simulink model "quadruped_2016"  (R2016a)
settings: Solver=ode23t  SolverMode=SingleTasking  StartTime=0.0  StopTime=8  RelTol=1e-3
values from neighbouring files (symbols this model uses):
  robot = Robot    [quadruped_sim_param.m]
undefined symbols (not defined in the file or in its folder): sigbuilder_block, X, Y, Z
undefined symbols (not defined in the file): plane
libraries: sm_lib x138, nesl_utility x66, simulink x24, Contact_Forces_Lib x12
(part 1 of 5)
settings Model: Creator=krzysiek  LastModifiedBy=krzysiek
settings SolverCC: ZeroCrossAlgorithm=Adaptive
settings DataIOCC: ReturnWorkspaceOutputs=on
settings DebuggingCC: IgnoredZcDiagnostic=none  SFUnexpectedBacktrackingDiag=error  SFNoUnconditionalDefaultTransitionDiag=error
settings SFSimCC: SimUseLocalCustomCode=on
settings RTWCC: RTWUseLocalCustomCode=on
settings GRTTargetCC: TargetLangStandard=C99 (ISO)  GeneratePreprocessorConditionals=Use local settings
settings ConfigComp: CovMetricSettings=dwe  CovHtmlReporting=off  CovSaveCumulativeToWorkspaceVar=off  CovSaveSingleToWorkspaceVar=off  CovExternalEMLEnable=on
settings DiagnosticsConfigSet: SimMechanicsRigidlyBoundBlock=none

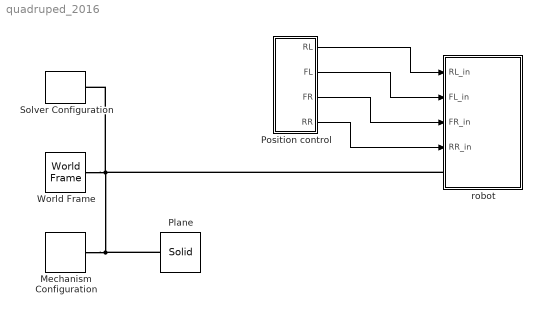
== system quadruped_2016 ==
  Mechanism Configuration : sm_lib/Utilities/Mechanism Configuration  UniformGravity=Constant  GravityVector=[0 0 -9.80665]  GravityUnits=m/s^2  LinearizationDelta=0.001
  "Plane " : sm_lib/Body Elements/Solid  GraphicAmbientColor=[0.15 0.15 0.15 1.0]  BasedOnType=Density  BrickDimensions=plane  BrickDimensionUnits=m  CenterOfMass=[0 0 0]  CenterOfMassUnits=m  GraphicDiffuseColor=[0.5 0.5 0.5]  Density=1000  DensityUnits=kg/m^3  DoExposeReferenceFrame=on  GraphicEmissiveColor=[0.0 0.0 0.0 1.0]  ExportEntireGeometry=off  SerializedFrames=<Frames/>  MarkerShape=Sphere  MarkerSize=10  GraphicType=FromGeometry  InertiaType=CalculateFromGeometry  Mass=1  MassUnits=kg  MomentsOfInertia=[1 1 1]  MomentsOfInertiaUnits=kg*m^2  GraphicOpacity=1.0  ProductsOfInertia=[0 0 0]  ProductsOfInertiaUnits=kg*m^2  GraphicShininess=75  GraphicSpecularColor=[0.5 0.5 0.5 1.0]  GraphicVisPropType=SimpleVisualProperties  GeometryShape=Brick
  Position control : Subsystem
  Solver Configuration : nesl_utility/Solver Configuration  PhysicalDomain=network_engine_domain  SubClassName=solver  LeftPortType=input  RightPortType=generic  Tones=[]  Harmonics=[]  SimulateNoise=off  Profile=off  UseLocalSampling=off  EnableSwitchedLinearOptims=on  FrequencyDomain=off  UseCCode=off  RelTol=0.001  AbsTol=1e-06  MinStep=1e-09  ToWorkspace=off  RevertToSquareIcSolve=off  NumHomotopyIterations=100  PhasorMode=off  PhasorModeNumHarmonics=1  DoDC=off  ResidualTolerance=1e-09  UseLocalSolver=off  LocalSolverChoice=NE_TRAPEZOIDAL_ADVANCER  LocalSolverSampleTime=0.1  DoFixedCost=off  MaxNonlinIter=3  MaxModeIter=2  LinearAlgebra=Sparse  EquationFormulation=NE_TIME_EF  DelaysMemoryBudget=1024  AutomaticFiltering=on  FilteringTimeConstant=0.001  PartitionStorageMethod=AS_NEEDED  PartitionMemoryBudget=1024  PartitionMethod=FAST
  World Frame : sm_lib/Frames and Transforms/World Frame
  robot : Subsystem
  wires:
  Position control/1(RL) -> robot/1(RL_in)
  Position control/2(FL) -> robot/2(FL_in)
  Position control/3(FR) -> robot/3(FR_in)
  Position control/4(RR) -> robot/4(RR_in)
  connections:
  World Frame/RConn1 -- Mechanism Configuration/RConn1 -- "Plane "/RConn1 -- robot/LConn1 -- Solver Configuration/RConn1

== system quadruped_2016/Position control ==
  Constant1 : Constant  Value=robot.FL.hip.joint.base_angle
  Constant2 : Constant  Value=robot.FR.hip.joint.base_angle
  Constant3 : Constant  Value=robot.RR.hip.joint.base_angle
  Constant6 : Constant  Value=robot.RL.hip.joint.base_angle
  Mux{1..4} (4 alike) : Mux  Inputs=3
  Signal Builder : Subsystem  Tag=STV Subsys  LoadFcn=sigbuilder_block('load');  StartFcn=sigbuilder_block('start');  StopFcn=sigbuilder_block('stop');  ClipboardFcn=sigbuilder_block('clipboard');  mask(Sigbuilder block){}
      mask help: Simulink:masks:SigbuilderBlock_MD
      mask init:
      | if ~strcmp(get_param(bdroot(gcbh),'SimulationStatus'),'stopped') tuvar = sigbuilder_block('maskInit'); end
      settings: CopyFcn=sigbuilder_block('copy');  DeleteFcn=sigbuilder_block('delete');  ModelCloseFcn=sigbuilder_block('modelClose');  PreSaveFcn=sigbuilder_block('preSave');  PauseFcn=sigbuilder_block('pause');  ContinueFcn=sigbuilder_block('continue');  NameChangeFcn=sigbuilder_block('namechange');  OpenFcn=sigbuilder_block('open',[1212.63 0 1212.63 628.421 ]);  CloseFcn=sigbuilder_block('close');
      mask Display: plot(0, 0, 100, 100,[2, 2, 32, 32, 2], [68, 8, 8, 68, 68],[32, 2], [38, 38], [32, 19, 2],[53, 60, 44], [32, 17, 17, 2],[16, 16, 31, 31]);txt = getActiveGroup(gcbh);text(2, 100, txt,'verticalAlignment', 'top');
  RL : Outport
  FL : Outport  Port=2
  FR : Outport  Port=3
  RR : Outport  Port=4
  wires:
  Mux2/1 -> RL/1
  Constant6/1 -> Mux2/3  "hip pos"
  Mux1/1 -> FL/1
  Constant1/1 -> Mux1/3  "hip pos"
  Mux3/1 -> FR/1
  Constant2/1 -> Mux3/3  "hip pos"
  Mux4/1 -> RR/1
  Constant3/1 -> Mux4/3  "hip pos"
  Signal Builder/1(Rx) -> Mux2/1, Mux4/1  "x"
  Signal Builder/2(Ry) -> Mux2/2, Mux4/2
  Signal Builder/3(Fx) -> Mux1/1, Mux3/1  "x"
  Signal Builder/4(Fy) -> Mux1/2, Mux3/2  "y"

== system quadruped_2016/robot ==
  RL_in : Inport
  FL_in : Inport  Port=2
  FR_in : Inport  Port=3
  RR_in : Inport  Port=4
  6-DOF Joint1 : sm_lib/Joints/6-DOF Joint  JointMode=Normal  SenseConstraintForce=off  SenseConstraintForceX=off  SenseConstraintForceY=off  SenseConstraintForceZ=off  SenseConstraintTorque=off  SenseConstraintTorqueX=off  SenseConstraintTorqueY=off  SenseConstraintTorqueZ=off  SenseTotalForce=off  SenseTotalForceX=off  SenseTotalForceY=off  SenseTotalForceZ=off  SenseTotalTorque=off  SenseTotalTorqueX=off  SenseTotalTorqueY=off  SenseTotalTorqueZ=off  CompositeWrenchDir=FollowerOnBase  CompositeWrenchFrame=BaseFrame  PxEquilibriumPosition=0  PxEquilibriumPositionUnits=m  PxSpringStiffness=0  PxSpringStiffnessUnits=N/m  PxDampingCoefficient=0  PxDampingCoefficientUnits=N/(m/s)  PxTorqueActuationMode=NoTorque  PxMotionActuationMode=ComputedMotion  PxSensePosition=off  PxSenseVelocity=off  PxSenseAcceleration=off  PxSenseTorqueForce=off  PxSenseLowerLimitTorqueForce=off  PxSenseUpperLimitTorqueForce=off  PxLowerLimitSpecify=off  PxLowerLimitBound=-1  PxLowerLimitBoundUnits=m  PxLowerLimitStiffness=1e6  PxLowerLimitStiffnessUnits=N/m  PxLowerLimitDamping=1e3  PxLowerLimitDampingUnits=N/(m/s)  PxLowerLimitTransitionRegionWidth=1e-4  PxLowerLimitTransitionRegionWidthUnits=m  PxUpperLimitSpecify=off  PxUpperLimitBound=1  PxUpperLimitBoundUnits=m  PxUpperLimitStiffness=1e6  PxUpperLimitStiffnessUnits=N/m  PxUpperLimitDamping=1e3  PxUpperLimitDampingUnits=N/(m/s)  PxUpperLimitTransitionRegionWidth=1e-4  PxUpperLimitTransitionRegionWidthUnits=m  PxPositionTargetSpecify=off  PxPositionTargetPriority=High  PxPositionTargetValue=0  PxPositionTargetValueUnits=m  PxVelocityTargetSpecify=off  PxVelocityTargetPriority=High  PxVelocityTargetValue=0  PxVelocityTargetValueUnits=m/s  PyEquilibriumPosition=0  PyEquilibriumPositionUnits=m  PySpringStiffness=0  PySpringStiffnessUnits=N/m  PyDampingCoefficient=0  PyDampingCoefficientUnits=N/(m/s)  PyTorqueActuationMode=NoTorque  PyMotionActuationMode=ComputedMotion  PySensePosition=off  PySenseVelocity=off  PySenseAcceleration=off  PySenseTorqueForce=off  PySenseLowerLimitTorqueForce=off  PySenseUpperLimitTorqueForce=off  PyLowerLimitSpecify=off  PyLowerLimitBound=-1  PyLowerLimitBoundUnits=m  PyLowerLimitStiffness=1e6  PyLowerLimitStiffnessUnits=N/m  PyLowerLimitDamping=1e3  PyLowerLimitDampingUnits=N/(m/s)  PyLowerLimitTransitionRegionWidth=1e-4  PyLowerLimitTransitionRegionWidthUnits=m  PyUpperLimitSpecify=off  PyUpperLimitBound=1  PyUpperLimitBoundUnits=m  PyUpperLimitStiffness=1e6  PyUpperLimitStiffnessUnits=N/m  PyUpperLimitDamping=1e3  PyUpperLimitDampingUnits=N/(m/s)  PyUpperLimitTransitionRegionWidth=1e-4  PyUpperLimitTransitionRegionWidthUnits=m  PyPositionTargetSpecify=off  PyPositionTargetPriority=High  PyPositionTargetValue=0  PyPositionTargetValueUnits=m  PyVelocityTargetSpecify=off  PyVelocityTargetPriority=High  PyVelocityTargetValue=0  PyVelocityTargetValueUnits=m/s  PzEquilibriumPosition=0  PzEquilibriumPositionUnits=m  PzSpringStiffness=0  PzSpringStiffnessUnits=N/m  PzDampingCoefficient=0  PzDampingCoefficientUnits=N/(m/s)  PzTorqueActuationMode=NoTorque  PzMotionActuationMode=ComputedMotion  PzSensePosition=off  PzSenseVelocity=off  PzSenseAcceleration=off  PzSenseTorqueForce=off  PzSenseLowerLimitTorqueForce=off  PzSenseUpperLimitTorqueForce=off  PzLowerLimitSpecify=off  PzLowerLimitBound=-1  PzLowerLimitBoundUnits=m  PzLowerLimitStiffness=1e6  PzLowerLimitStiffnessUnits=N/m  PzLowerLimitDamping=1e3  PzLowerLimitDampingUnits=N/(m/s)  PzLowerLimitTransitionRegionWidth=1e-4  PzLowerLimitTransitionRegionWidthUnits=m  PzUpperLimitSpecify=off  PzUpperLimitBound=1  PzUpperLimitBoundUnits=m  PzUpperLimitStiffness=1e6  PzUpperLimitStiffnessUnits=N/m  PzUpperLimitDamping=1e3  PzUpperLimitDampingUnits=N/(m/s)  PzUpperLimitTransitionRegionWidth=1e-4  PzUpperLimitTransitionRegionWidthUnits=m  PzPositionTargetSpecify=off  PzPositionTargetPriority=High  PzPositionTargetValue=0  PzPositionTargetValueUnits=m  PzVelocityTargetSpecify=off  PzVelocityTargetPriority=High  PzVelocityTargetValue=0  PzVelocityTargetValueUnits=m/s  SphDefPosRotationMethod=None  SphDefPosRotationAngleUnits=deg  SphDefPosRotationStandardAxis=+Z  SphDefPosRotationAngle=0.0  SphDefPosRotationArbitraryAxis=[0 0 1]  SphDefPosFollAlignAxisA=+X  SphDefPosBaseAlignAxisA=+Y  SphDefPosFollAlignAxisB=+Y  SphDefPosBaseAlignAxisB=+Z  SphDefPosRotationSequenceAxes=FollowerAxes  SphDefPosRotationSequence=XYX  SphDefPosRotationSequenceAngles=[0 0 0]  SphDefPosRotationSequenceAnglesUnits=deg  SphDefPosRotationMatrix=[1 0 0; 0 1 0; 0 0 1]  SphEqPosRotationMethod=None  SphEqPosRotationAngleUnits=deg  SphEqPosRotationStandardAxis=+Z  SphEqPosRotationAngle=0.0  SphEqPosRotationArbitraryAxis=[0 0 1]  SphEqPosFollAlignAxisA=+X  SphEqPosBaseAlignAxisA=+Y  SphEqPosFollAlignAxisB=+Y  SphEqPosBaseAlignAxisB=+Z  SphEqPosRotationSequenceAxes=FollowerAxes  SphEqPosRotationSequence=XYX  SphEqPosRotationSequenceAngles=[0 0 0]  SphEqPosRotationSequenceAnglesUnits=deg  SphEqPosRotationMatrix=[1 0 0; 0 1 0; 0 0 1]  SphSpringStiffness=0  SphSpringStiffnessUnits=N*m/deg  SphDampingCoefficient=0  SphDampingCoefficientUnits=N*m/(deg/s)  SphActuateTorqueX=off  SphActuateTorqueY=off  SphActuateTorqueZ=off  SphActuateTorque=off  SphTorqueActuationMode=NoTorque  SphMotionActuationMode=ComputedMotion  SphActuationFrame=BaseFrame  SphSensePosition=off  SphSenseVelocityX=off  SphSenseVelocityY=off  SphSenseVelocityZ=off  SphSenseVelocity=off  SphSenseAccelerationX=off  SphSenseAccelerationY=off  SphSenseAccelerationZ=off  SphSenseAcceleration=off  SphSenseTorqueX=off  SphSenseTorqueY=off  SphSenseTorqueZ=off  SphSenseTorqueForce=off  SphSenseLowerLimitTorqueMag=off  SphSenseUpperLimitTorqueMag=off  SphSensingFrame=BaseFrame  SphLowerLimitSpecify=off  SphLowerLimitBound=15  SphLowerLimitBoundUnits=deg  SphLowerLimitStiffness=1e4  SphLowerLimitStiffnessUnits=N*m/deg  SphLowerLimitDamping=10  SphLowerLimitDampingUnits=N*m/(deg/s)  SphLowerLimitTransitionRegionWidth=0.1  SphLowerLimitTransitionRegionWidthUnits=deg  SphUpperLimitSpecify=off  SphUpperLimitBound=45  SphUpperLimitBoundUnits=deg  SphUpperLimitStiffness=1e4  SphUpperLimitStiffnessUnits=N*m/deg  SphUpperLimitDamping=10  SphUpperLimitDampingUnits=N*m/(deg/s)  SphUpperLimitTransitionRegionWidth=0.1  SphUpperLimitTransitionRegionWidthUnits=deg  SphPositionTargetRotationMethod=None  SphPositionTargetRotationAngleUnits=deg  SphPositionTargetRotationStandardAxis=+Z  SphPositionTargetRotationAngle=0.0  SphPositionTargetRotationArbitraryAxis=[0 0 1]  SphPositionTargetFollAlignAxisA=+X  SphPositionTargetBaseAlignAxisA=+Y  SphPositionTargetFollAlignAxisB=+Y  SphPositionTargetBaseAlignAxisB=+Z  SphPositionTargetRotationSequenceAxes=FollowerAxes  SphPositionTargetRotationSequence=XYX  SphPositionTargetRotationSequenceAngles=[0 0 0]  SphPositionTargetRotationSequenceAnglesUnits=deg  SphPositionTargetRotationMatrix=[1 0 0; 0 1 0; 0 0 1]  SphPositionTargetSpecify=off  SphPositionTargetPriority=High  SphVelocityTargetValue=[0 0 0]  SphVelocityTargetValueUnits=deg/s  SphVelocityTargetSpecify=off  SphVelocityTargetPriority=High  SphVelocityTargetInFollowerFrame=on
  FL : Subsystem  mask{Leg=robot.FL, plane_dim=plane}
  FR : Subsystem  mask{Leg=robot.FR, plane_dim=plane}
  RL : Subsystem  mask{Leg=robot.RL, plane_dim=plane}
  RR : Subsystem  mask{Leg=robot.RR, plane_dim=plane}
  Rigid Transform : sm_lib/Frames and Transforms/Rigid Transform  TranslationMethod=StandardAxis  TranslationStandardOffset=270  TranslationLengthUnit=mm  TranslationStandardAxis=+Z  TranslationCartesianOffset=[0 0 0]  TranslationROffset=0  TranslationROffsetUnits=m  TranslationZOffset=0  TranslationZOffsetUnits=m  TranslationThetaOffset=0  TranslationThetaOffsetUnits=deg  RotationMethod=None  RotationAngleUnits=deg  RotationStandardAxis=+Z  RotationAngle=0.0  RotationArbitraryAxis=[0 0 1]  FollAlignAxisA=+X  BaseAlignAxisA=+Y  FollAlignAxisB=+Y  BaseAlignAxisB=+Z  RotationSequenceAxes=FollowerAxes  RotationSequence=XYX  RotationSequenceAngles=[0 0 0]  RotationSequenceAnglesUnits=deg  RotationMatrix=[1 0 0; 0 1 0; 0 0 1]
  Terminator{,1..4} (5 alike) : Terminator
  robot body : Subsystem  mask{robot=robot}
  plane : PMIOPort  Side=Left
  wires:
  RL_in/1 -> RL/1(pos)
  robot body/1(p) -> Terminator4/1
  RL/1(p) -> Terminator1/1
  RR/1(p) -> Terminator/1
  FR_in/1 -> FR/1(pos)
  RR_in/1 -> RR/1(pos)
  FL/1(p) -> Terminator2/1
  FR/1(p) -> Terminator3/1
  FL_in/1 -> FL/1(pos)
  connections:
  6-DOF Joint1/LConn1 -- Rigid Transform/RConn1
  FR/LConn1 -- robot body/RConn2
  RR/LConn1 -- robot body/LConn4
  6-DOF Joint1/RConn1 -- robot body/LConn2
  FL/LConn1 -- robot body/RConn1
  RL/LConn1 -- robot body/LConn1
  FR/RConn1 -- robot body/LConn3 -- FL/RConn1 -- RL/RConn1 -- Rigid Transform/LConn1 -- plane/RConn1 -- RR/RConn1

== system quadruped_2016/Position control/Signal Builder ==
  Demux : Demux  Tag=STV Demux
  FromWs : FromWorkspace  Tag=STV FromWs  VariableName=tuvar  SampleTime=0
      SigBuilderData=|
      | common.afterFinalStr = 'Extrapolate'
      | common.sampleTime = 0
      | dataSet.timeRange = [0 10]
      | dataSet.name = 'Group 1'
      | sbobj.Groups.Name = 'Group 1'
      | sbobj.Groups.Signals(1).Name = 'Rx'
      | sbobj.Groups.Signals(1).XData = [0 0.88 0.88 1.43 1.43 10]
      | sbobj.Groups.Signals(1).YData = [-6 -10 -54 -242 -10 -12]
      | sbobj.Groups.Signals(2).Name = 'Ry'
      | sbobj.Groups.Signals(2).XData = [0 0.85 0.85 1.36 1.36 10]
      | sbobj.Groups.Signals(2).YData = [100 100 145 325 150 150]
      | sbobj.Groups.Signals(3).Name = 'Fx'
      | sbobj.Groups.Signals(3).XData = [0 0.8 0.8 1.35 1.35 10]
      | sbobj.Groups.Signals(3).YData = [-70 -70 -71 -142 -14 -25]
      | sbobj.Groups.Signals(4).Name = 'Fy'
      | sbobj.Groups.Signals(4).XData = [0 0.74 0.74 1.29 1.29 10]
      | sbobj.Groups.Signals(4).YData = [100 100 90 315 135 150]
  Rx : Outport  Tag=STV Outport
  Ry : Outport  Tag=STV Outport  Port=2
  Fx : Outport  Tag=STV Outport  Port=3
  Fy : Outport  Tag=STV Outport  Port=4
  wires:
  FromWs/1 -> Demux/1
  Demux/1 -> Rx/1
  Demux/2 -> Ry/1
  Demux/3 -> Fx/1
  Demux/4 -> Fy/1

== system quadruped_2016/robot/FL ==
  pos : Inport
  Bus Creator : BusCreator  Inputs=2
  Demux : Demux  Outputs=3
  "Inverse Kinematics " : Subsystem
  hip : Subsystem  mask{Hip=Leg.hip}
  leg : Subsystem
  plane : PMIOPort  Side=Right
  B : PMIOPort  Port=2  Side=Left
  p : Outport
  wires:
  Demux/3 -> hip/1(pos)  "hip pos"
  leg/1(p) -> Bus Creator/2  "leg"
  Bus Creator/1 -> p/1
  pos/1 -> Demux/1
  Demux/1 -> "Inverse Kinematics "/1(x)  "x"
  Demux/2 -> "Inverse Kinematics "/2(y)  "y"
  "Inverse Kinematics "/1(S) -> leg/1(up pos)
  "Inverse Kinematics "/2(E) -> leg/2(lo pos)
  hip/1(p) -> Bus Creator/1  "hip"
  connections:
  leg/LConn1 -- hip/RConn1
  hip/RConn2 -- plane/RConn1 -- leg/RConn1
  hip/LConn1 -- B/RConn1

== system quadruped_2016/robot/FR ==
  pos : Inport
  Bus Creator : BusCreator  Inputs=2
  Demux : Demux  Outputs=3
  "Inverse Kinematics " : Subsystem
  hip : Subsystem  mask{Hip=Leg.hip}
  leg : Subsystem
  plane : PMIOPort  Side=Right
  B : PMIOPort  Port=2  Side=Left
  p : Outport
  wires:
  Demux/3 -> hip/1(pos)  "hip pos"
  leg/1(p) -> Bus Creator/2  "leg"
  Bus Creator/1 -> p/1
  pos/1 -> Demux/1
  Demux/1 -> "Inverse Kinematics "/1(x)  "x"
  Demux/2 -> "Inverse Kinematics "/2(y)  "y"
  "Inverse Kinematics "/1(S) -> leg/1(up pos)
  "Inverse Kinematics "/2(E) -> leg/2(lo pos)
  hip/1(p) -> Bus Creator/1  "hip"
  connections:
  leg/LConn1 -- hip/RConn1
  hip/RConn2 -- plane/RConn1 -- leg/RConn1
  hip/LConn1 -- B/RConn1

== system quadruped_2016/robot/RL ==
  pos : Inport
  Bus Creator : BusCreator  Inputs=2
  Demux : Demux  Outputs=3
  "Inverse Kinematics " : Subsystem
  hip : Subsystem  mask{Hip=Leg.hip}
  leg : Subsystem
  plane : PMIOPort  Side=Right
  B : PMIOPort  Port=2  Side=Left
  p : Outport
  wires:
  Demux/3 -> hip/1(pos)  "hip pos"
  leg/1(p) -> Bus Creator/2  "leg"
  Bus Creator/1 -> p/1
  pos/1 -> Demux/1
  Demux/1 -> "Inverse Kinematics "/1(x)  "x"
  Demux/2 -> "Inverse Kinematics "/2(y)  "y"
  "Inverse Kinematics "/1(S) -> leg/1(up pos)
  "Inverse Kinematics "/2(E) -> leg/2(lo pos)
  hip/1(p) -> Bus Creator/1  "hip"
  connections:
  leg/LConn1 -- hip/RConn1
  hip/RConn2 -- plane/RConn1 -- leg/RConn1
  hip/LConn1 -- B/RConn1

== system quadruped_2016/robot/RR ==
  pos : Inport
  Bus Creator : BusCreator  Inputs=2
  Demux : Demux  Outputs=3
  "Inverse Kinematics " : Subsystem
  hip : Subsystem  mask{Hip=Leg.hip}
  leg : Subsystem
  plane : PMIOPort  Side=Right
  B : PMIOPort  Port=2  Side=Left
  p : Outport
  wires:
  Demux/3 -> hip/1(pos)  "hip pos"
  leg/1(p) -> Bus Creator/2  "leg"
  Bus Creator/1 -> p/1
  pos/1 -> Demux/1
  Demux/1 -> "Inverse Kinematics "/1(x)  "x"
  Demux/2 -> "Inverse Kinematics "/2(y)  "y"
  "Inverse Kinematics "/1(S) -> leg/1(up pos)
  "Inverse Kinematics "/2(E) -> leg/2(lo pos)
  hip/1(p) -> Bus Creator/1  "hip"
  connections:
  leg/LConn1 -- hip/RConn1
  hip/RConn2 -- plane/RConn1 -- leg/RConn1
  hip/LConn1 -- B/RConn1

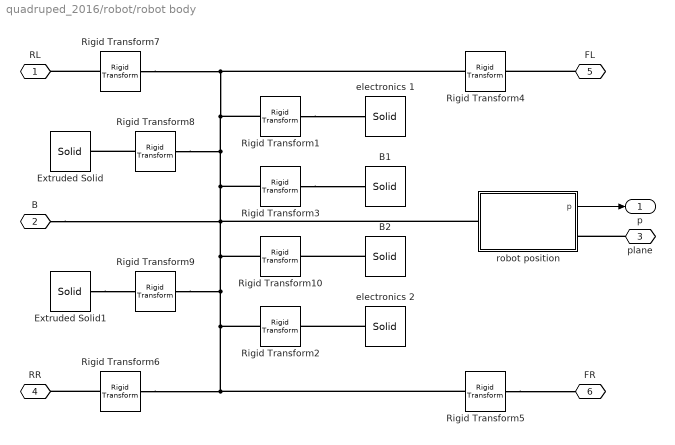
== system quadruped_2016/robot/robot body ==
  B1 : sm_lib/Body Elements/Solid  GraphicAmbientColor=[0.15 0.15 0.15 1.0]  BasedOnType=Mass  BrickDimensions=robot.b1.dimension  BrickDimensionUnits=mm  CenterOfMass=[0 0 0]  CenterOfMassUnits=m  GraphicDiffuseColor=robot.b1.color  Density=robot.b1.density  DensityUnits=kg/m^3  DoExposeReferenceFrame=on  GraphicEmissiveColor=[0.0 0.0 0.0 1.0]  ExportEntireGeometry=off  SerializedFrames=<Frames/>  MarkerShape=Sphere  MarkerSize=10  GraphicType=FromGeometry  InertiaType=CalculateFromGeometry  Mass=robot.b1.mass  MassUnits=g  MomentsOfInertia=[1 1 1]  MomentsOfInertiaUnits=kg*m^2  GraphicOpacity=1.0  ProductsOfInertia=[0 0 0]  ProductsOfInertiaUnits=kg*m^2  GraphicShininess=75  GraphicSpecularColor=[0.5 0.5 0.5 1.0]  GraphicVisPropType=SimpleVisualProperties  GeometryShape=Brick
  B2 : sm_lib/Body Elements/Solid  GraphicAmbientColor=[0.15 0.15 0.15 1.0]  BasedOnType=Mass  BrickDimensions=robot.b2.dimension  BrickDimensionUnits=mm  CenterOfMass=[0 0 0]  CenterOfMassUnits=m  GraphicDiffuseColor=robot.b1.color  Density=robot.b2.density  DensityUnits=kg/m^3  DoExposeReferenceFrame=on  GraphicEmissiveColor=[0.0 0.0 0.0 1.0]  ExportEntireGeometry=off  SerializedFrames=<Frames/>  MarkerShape=Sphere  MarkerSize=10  GraphicType=FromGeometry  InertiaType=CalculateFromGeometry  Mass=robot.b1.mass  MassUnits=g  MomentsOfInertia=[1 1 1]  MomentsOfInertiaUnits=kg*m^2  GraphicOpacity=1.0  ProductsOfInertia=[0 0 0]  ProductsOfInertiaUnits=kg*m^2  GraphicShininess=75  GraphicSpecularColor=[0.5 0.5 0.5 1.0]  GraphicVisPropType=SimpleVisualProperties  GeometryShape=Brick
  Extruded Solid : sm_lib/Body Elements/Solid  GraphicAmbientColor=[0.15 0.15 0.15 1.0]  BasedOnType=Mass  CenterOfMass=[0 0 0]  CenterOfMassUnits=m  GraphicDiffuseColor=robot.enclosure.color  ExtrusionCrossSection=[1 1; -1 1; -1 -1; 1 -1]  ExtrusionCrossSectionUnits=m  Density=robot.enclosure.density  DensityUnits=kg/m^3  DoExposeReferenceFrame=on  GraphicEmissiveColor=[0.0 0.0 0.0 1.0]  ExportEntireGeometry=off  ExtrusionLength=robot.enclosure.dimension(3)  ExtrusionLengthUnits=mm  ExtrusionType=Regular  SerializedFrames=<Frames/>  MarkerShape=Sphere  MarkerSize=10  GraphicType=FromGeometry  InertiaType=CalculateFromGeometry  Mass=robot.enclosure.mass  MassUnits=g  MomentsOfInertia=[1 1 1]  MomentsOfInertiaUnits=kg*m^2  PolygonNumSides=6  GraphicOpacity=robot.enclosure.opacity  PolygonOuterRadius=robot.enclosure.dimension(1)  PolygonOuterRadiusUnits=mm  ProductsOfInertia=[0 0 0]  ProductsOfInertiaUnits=kg*m^2  GraphicShininess=75  GraphicSpecularColor=[0.5 0.5 0.5 1.0]  GraphicVisPropType=SimpleVisualProperties  GeometryShape=RegularExtrusion
  Extruded Solid1 : sm_lib/Body Elements/Solid  GraphicAmbientColor=[0.15 0.15 0.15 1.0]  BasedOnType=Mass  CenterOfMass=[0 0 0]  CenterOfMassUnits=m  GraphicDiffuseColor=robot.enclosure.color  ExtrusionCrossSection=[1 1; -1 1; -1 -1; 1 -1]  ExtrusionCrossSectionUnits=m  Density=robot.enclosure.density  DensityUnits=kg/m^3  DoExposeReferenceFrame=on  GraphicEmissiveColor=[0.0 0.0 0.0 1.0]  ExportEntireGeometry=off  ExtrusionLength=robot.enclosure.dimension(3)  ExtrusionLengthUnits=mm  ExtrusionType=Regular  SerializedFrames=<Frames/>  MarkerShape=Sphere  MarkerSize=10  GraphicType=FromGeometry  InertiaType=CalculateFromGeometry  Mass=robot.enclosure.mass  MassUnits=g  MomentsOfInertia=[1 1 1]  MomentsOfInertiaUnits=kg*m^2  PolygonNumSides=6  GraphicOpacity=robot.enclosure.opacity  PolygonOuterRadius=robot.enclosure.dimension(1)  PolygonOuterRadiusUnits=mm  ProductsOfInertia=[0 0 0]  ProductsOfInertiaUnits=kg*m^2  GraphicShininess=75  GraphicSpecularColor=[0.5 0.5 0.5 1.0]  GraphicVisPropType=SimpleVisualProperties  GeometryShape=RegularExtrusion
  Rigid Transform1 : sm_lib/Frames and Transforms/Rigid Transform  TranslationMethod=Cartesian  TranslationStandardOffset=0  TranslationLengthUnit=mm  TranslationStandardAxis=+Z  TranslationCartesianOffset=robot.odrv_l.position  TranslationROffset=0  TranslationROffsetUnits=m  TranslationZOffset=0  TranslationZOffsetUnits=m  TranslationThetaOffset=0  TranslationThetaOffsetUnits=deg  RotationMethod=StandardAxis  RotationAngleUnits=deg  RotationStandardAxis=+X  RotationAngle=90  RotationArbitraryAxis=[0 0 1]  FollAlignAxisA=+X  BaseAlignAxisA=+Y  FollAlignAxisB=+Y  BaseAlignAxisB=+Z  RotationSequenceAxes=FollowerAxes  RotationSequence=XYX  RotationSequenceAngles=[0 0 0]  RotationSequenceAnglesUnits=deg  RotationMatrix=[1 0 0; 0 1 0; 0 0 1]
  Rigid Transform10 : sm_lib/Frames and Transforms/Rigid Transform  TranslationMethod=Cartesian  TranslationStandardOffset=0  TranslationLengthUnit=mm  TranslationStandardAxis=+Z  TranslationCartesianOffset=robot.b2.position  TranslationROffset=0  TranslationROffsetUnits=m  TranslationZOffset=0  TranslationZOffsetUnits=m  TranslationThetaOffset=0  TranslationThetaOffsetUnits=deg  RotationMethod=StandardAxis  RotationAngleUnits=deg  RotationStandardAxis=+X  RotationAngle=90  RotationArbitraryAxis=[0 0 1]  FollAlignAxisA=+X  BaseAlignAxisA=+Y  FollAlignAxisB=+Y  BaseAlignAxisB=+Z  RotationSequenceAxes=FollowerAxes  RotationSequence=XYX  RotationSequenceAngles=[0 0 0]  RotationSequenceAnglesUnits=deg  RotationMatrix=[1 0 0; 0 1 0; 0 0 1]
  Rigid Transform2 : sm_lib/Frames and Transforms/Rigid Transform  TranslationMethod=Cartesian  TranslationStandardOffset=0  TranslationLengthUnit=mm  TranslationStandardAxis=+Z  TranslationCartesianOffset=robot.odrv_r.position  TranslationROffset=0  TranslationROffsetUnits=m  TranslationZOffset=0  TranslationZOffsetUnits=m  TranslationThetaOffset=0  TranslationThetaOffsetUnits=deg  RotationMethod=StandardAxis  RotationAngleUnits=deg  RotationStandardAxis=+X  RotationAngle=90  RotationArbitraryAxis=[0 0 1]  FollAlignAxisA=+X  BaseAlignAxisA=+Y  FollAlignAxisB=+Y  BaseAlignAxisB=+Z  RotationSequenceAxes=FollowerAxes  RotationSequence=XYX  RotationSequenceAngles=[0 0 0]  RotationSequenceAnglesUnits=deg  RotationMatrix=[1 0 0; 0 1 0; 0 0 1]
  Rigid Transform3 : sm_lib/Frames and Transforms/Rigid Transform  TranslationMethod=Cartesian  TranslationStandardOffset=0  TranslationLengthUnit=mm  TranslationStandardAxis=+Z  TranslationCartesianOffset=robot.b1.position  TranslationROffset=0  TranslationROffsetUnits=m  TranslationZOffset=0  TranslationZOffsetUnits=m  TranslationThetaOffset=0  TranslationThetaOffsetUnits=deg  RotationMethod=StandardAxis  RotationAngleUnits=deg  RotationStandardAxis=+X  RotationAngle=90  RotationArbitraryAxis=[0 0 1]  FollAlignAxisA=+X  BaseAlignAxisA=+Y  FollAlignAxisB=+Y  BaseAlignAxisB=+Z  RotationSequenceAxes=FollowerAxes  RotationSequence=XYX  RotationSequenceAngles=[0 0 0]  RotationSequenceAnglesUnits=deg  RotationMatrix=[1 0 0; 0 1 0; 0 0 1]
  Rigid Transform4 : sm_lib/Frames and Transforms/Rigid Transform  TranslationMethod=Cartesian  TranslationStandardOffset=0  TranslationLengthUnit=mm  TranslationStandardAxis=+Z  TranslationCartesianOffset=[-robot.body.dimension(1)/2, robot.body.dimension(2)/2, 0]  TranslationROffset=0  TranslationROffsetUnits=m  TranslationZOffset=0  TranslationZOffsetUnits=m  TranslationThetaOffset=0  TranslationThetaOffsetUnits=deg  RotationMethod=RotationSequence  RotationAngleUnits=deg  RotationStandardAxis=+Z  RotationAngle=0.0  RotationArbitraryAxis=[0 0 1]  FollAlignAxisA=+X  BaseAlignAxisA=+Y  FollAlignAxisB=+Y  BaseAlignAxisB=+Z  RotationSequenceAxes=FollowerAxes  RotationSequence=XYZ  RotationSequenceAngles=[-90 0 180]  RotationSequenceAnglesUnits=deg  RotationMatrix=[1 0 0; 0 1 0; 0 0 1]
  Rigid Transform5 : sm_lib/Frames and Transforms/Rigid Transform  TranslationMethod=Cartesian  TranslationStandardOffset=0  TranslationLengthUnit=mm  TranslationStandardAxis=+Z  TranslationCartesianOffset=[robot.body.dimension(1)/2, robot.body.dimension(2)/2, 0]  TranslationROffset=0  TranslationROffsetUnits=m  TranslationZOffset=0  TranslationZOffsetUnits=m  TranslationThetaOffset=0  TranslationThetaOffsetUnits=deg  RotationMethod=RotationSequence  RotationAngleUnits=deg  RotationStandardAxis=+Z  RotationAngle=0.0  RotationArbitraryAxis=[0 0 1]  FollAlignAxisA=+X  BaseAlignAxisA=+Y  FollAlignAxisB=+Y  BaseAlignAxisB=+Z  RotationSequenceAxes=FollowerAxes  RotationSequence=XYZ  RotationSequenceAngles=[-90 0 180]  RotationSequenceAnglesUnits=deg  RotationMatrix=[1 0 0; 0 1 0; 0 0 1]
  Rigid Transform6 : sm_lib/Frames and Transforms/Rigid Transform  TranslationMethod=Cartesian  TranslationStandardOffset=0  TranslationLengthUnit=mm  TranslationStandardAxis=+Z  TranslationCartesianOffset=[robot.body.dimension(1)/2, -robot.body.dimension(2)/2, 0]  TranslationROffset=0  TranslationROffsetUnits=m  TranslationZOffset=0  TranslationZOffsetUnits=m  TranslationThetaOffset=0  TranslationThetaOffsetUnits=deg  RotationMethod=RotationSequence  RotationAngleUnits=deg  RotationStandardAxis=+Z  RotationAngle=90  RotationArbitraryAxis=[0 0 1]  FollAlignAxisA=+X  BaseAlignAxisA=+Y  FollAlignAxisB=+Y  BaseAlignAxisB=+Z  RotationSequenceAxes=FollowerAxes  RotationSequence=XYZ  RotationSequenceAngles=[-90 0 180]  RotationSequenceAnglesUnits=deg  RotationMatrix=[1 0 0; 0 1 0; 0 0 1]
  Rigid Transform7 : sm_lib/Frames and Transforms/Rigid Transform  TranslationMethod=Cartesian  TranslationStandardOffset=0  TranslationLengthUnit=mm  TranslationStandardAxis=+Z  TranslationCartesianOffset=[-robot.body.dimension(1)/2, -robot.body.dimension(2)/2, 0]  TranslationROffset=0  TranslationROffsetUnits=m  TranslationZOffset=0  TranslationZOffsetUnits=m  TranslationThetaOffset=0  TranslationThetaOffsetUnits=deg  RotationMethod=RotationSequence  RotationAngleUnits=deg  RotationStandardAxis=+Z  RotationAngle=0.0  RotationArbitraryAxis=[0 0 1]  FollAlignAxisA=+X  BaseAlignAxisA=+Y  FollAlignAxisB=+Y  BaseAlignAxisB=+Z  RotationSequenceAxes=FollowerAxes  RotationSequence=XYZ  RotationSequenceAngles=[90 180 0]  RotationSequenceAnglesUnits=deg  RotationMatrix=[1 0 0; 0 1 0; 0 0 1]
  Rigid Transform8 : sm_lib/Frames and Transforms/Rigid Transform  TranslationMethod=Cartesian  TranslationStandardOffset=0  TranslationLengthUnit=mm  TranslationStandardAxis=+Z  TranslationCartesianOffset=robot.enclosure.position  TranslationROffset=0  TranslationROffsetUnits=m  TranslationZOffset=0  TranslationZOffsetUnits=m  TranslationThetaOffset=0  TranslationThetaOffsetUnits=deg  RotationMethod=StandardAxis  RotationAngleUnits=deg  RotationStandardAxis=+X  RotationAngle=90  RotationArbitraryAxis=[0 0 1]  FollAlignAxisA=+X  BaseAlignAxisA=+Y  FollAlignAxisB=+Y  BaseAlignAxisB=+Z  RotationSequenceAxes=FollowerAxes  RotationSequence=XYX  RotationSequenceAngles=[0 0 0]  RotationSequenceAnglesUnits=deg  RotationMatrix=[1 0 0; 0 1 0; 0 0 1]
  Rigid Transform9 : sm_lib/Frames and Transforms/Rigid Transform  TranslationMethod=Cartesian  TranslationStandardOffset=0  TranslationLengthUnit=mm  TranslationStandardAxis=+Z  TranslationCartesianOffset=-robot.enclosure.position  TranslationROffset=0  TranslationROffsetUnits=m  TranslationZOffset=0  TranslationZOffsetUnits=m  TranslationThetaOffset=0  TranslationThetaOffsetUnits=deg  RotationMethod=StandardAxis  RotationAngleUnits=deg  RotationStandardAxis=+X  RotationAngle=90  RotationArbitraryAxis=[0 0 1]  FollAlignAxisA=+X  BaseAlignAxisA=+Y  FollAlignAxisB=+Y  BaseAlignAxisB=+Z  RotationSequenceAxes=FollowerAxes  RotationSequence=XYX  RotationSequenceAngles=[0 0 0]  RotationSequenceAnglesUnits=deg  RotationMatrix=[1 0 0; 0 1 0; 0 0 1]
  electronics 1 : sm_lib/Body Elements/Solid  GraphicAmbientColor=[0.15 0.15 0.15 1.0]  BasedOnType=Mass  BrickDimensions=robot.odrv_l.dimension  BrickDimensionUnits=mm  CenterOfMass=[0 0 0]  CenterOfMassUnits=m  GraphicDiffuseColor=robot.odrv_l.color  Density=1000  DensityUnits=kg/m^3  DoExposeReferenceFrame=on  GraphicEmissiveColor=[0.0 0.0 0.0 1.0]  ExportEntireGeometry=off  SerializedFrames=<Frames/>  MarkerShape=Sphere  MarkerSize=10  GraphicType=FromGeometry  InertiaType=CalculateFromGeometry  Mass=robot.odrv_l.mass  MassUnits=g  MomentsOfInertia=[1 1 1]  MomentsOfInertiaUnits=kg*m^2  GraphicOpacity=1.0  ProductsOfInertia=[0 0 0]  ProductsOfInertiaUnits=kg*m^2  GraphicShininess=75  GraphicSpecularColor=[0.5 0.5 0.5 1.0]  GraphicVisPropType=SimpleVisualProperties  GeometryShape=Brick
  electronics 2 : sm_lib/Body Elements/Solid  GraphicAmbientColor=[0.15 0.15 0.15 1.0]  BasedOnType=Mass  BrickDimensions=robot.odrv_r.dimension  BrickDimensionUnits=mm  CenterOfMass=[0 0 0]  CenterOfMassUnits=m  GraphicDiffuseColor=robot.odrv_r.color  Density=1000  DensityUnits=kg/m^3  DoExposeReferenceFrame=on  GraphicEmissiveColor=[0.0 0.0 0.0 1.0]  ExportEntireGeometry=off  SerializedFrames=<Frames/>  MarkerShape=Sphere  MarkerSize=10  GraphicType=FromGeometry  InertiaType=CalculateFromGeometry  Mass=robot.odrv_r.mass  MassUnits=g  MomentsOfInertia=[1 1 1]  MomentsOfInertiaUnits=kg*m^2  GraphicOpacity=1.0  ProductsOfInertia=[0 0 0]  ProductsOfInertiaUnits=kg*m^2  GraphicShininess=75  GraphicSpecularColor=[0.5 0.5 0.5 1.0]  GraphicVisPropType=SimpleVisualProperties  GeometryShape=Brick
  robot position : Subsystem
  RL : PMIOPort  Side=Left
  B : PMIOPort  Port=2  Side=Left
  "plane " : PMIOPort  Port=3  Side=Left
  RR : PMIOPort  Port=4  Side=Left
  FL : PMIOPort  Port=5  Side=Right
  FR : PMIOPort  Port=6  Side=Right
  p : Outport
  wires:
  robot position/1(p) -> p/1
  connections:
  B2/RConn1 -- Rigid Transform10/RConn1
  Rigid Transform3/RConn1 -- B1/RConn1
  Rigid Transform1/RConn1 -- electronics 1/RConn1
  electronics 2/RConn1 -- Rigid Transform2/RConn1
  Rigid Transform3/LConn1 -- B/RConn1 -- robot position/LConn1 -- Rigid Transform10/LConn1 -- Rigid Transform2/LConn1 -- Rigid Transform5/LConn1 -- Rigid Transform6/LConn1 -- Rigid Transform9/LConn1 -- Rigid Transform8/LConn1 -- Rigid Transform1/LConn1 -- Rigid Transform7/LConn1 -- Rigid Transform4/LConn1
  Rigid Transform6/RConn1 -- RR/RConn1
  Rigid Transform7/RConn1 -- RL/RConn1
  FL/RConn1 -- Rigid Transform4/RConn1
  Rigid Transform5/RConn1 -- FR/RConn1
  Rigid Transform8/RConn1 -- Extruded Solid/RConn1
  Extruded Solid1/RConn1 -- Rigid Transform9/RConn1
  "plane "/RConn1 -- robot position/RConn1

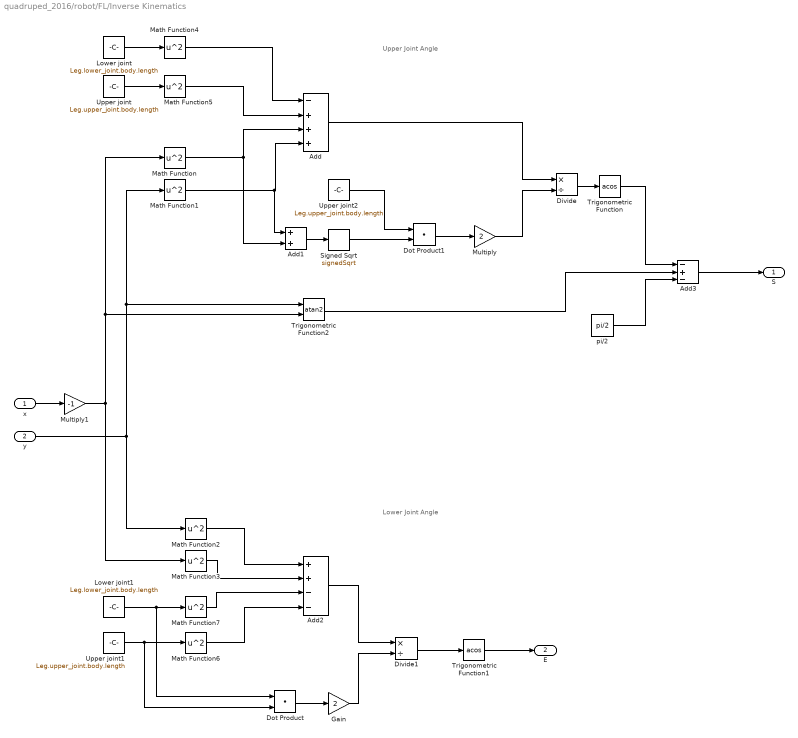
== system quadruped_2016/robot/FL/Inverse Kinematics  ==
  note: Upper Joint Angle
  note: Lower Joint Angle
  x : Inport
  y : Inport  Port=2
  Add : Sum  Inputs=-+++
  Add1 : Sum
  Add2 : Sum  Inputs=++--
  Add3 : Sum  Inputs=-+-
  Divide : Product  Inputs=*/
  Divide1 : Product  Inputs=*/
  Dot Product : DotProduct  InputSameDT=on  OutDataTypeStr=Inherit: Inherit via internal rule
  Dot Product1 : DotProduct  InputSameDT=on  OutDataTypeStr=Inherit: Inherit via internal rule
  Gain : Gain  Gain=2
  Lower joint : Constant  Value=Leg.lower_joint.body.length
  Lower joint1 : Constant  Value=Leg.lower_joint.body.length
  Math Function{,1..7} (8 alike) : Math  Operator=square  SaturateOnIntegerOverflow=on
  Multiply : Gain  Gain=2
  Multiply1 : Gain  Gain=-1
  Signed Sqrt : Sqrt  Operator=signedSqrt  SaturateOnIntegerOverflow=on
  Trigonometric Function : Trigonometry  Operator=acos
  Trigonometric Function1 : Trigonometry  Operator=acos
  Trigonometric Function2 : Trigonometry  Operator=atan2
  Upper joint : Constant  Value=Leg.upper_joint.body.length
  Upper joint1 : Constant  Value=Leg.upper_joint.body.length
  Upper joint2 : Constant  Value=Leg.upper_joint.body.length
  pi/2 : Constant  Value=pi/2
  S : Outport
  E : Outport  Port=2
  wires:
  y/1 -> Trigonometric Function2/1, Math Function1/1, Math Function2/1
  Lower joint/1 -> Math Function4/1
  Upper joint/1 -> Math Function5/1
  Math Function/1 -> Add1/2, Add/3
  Math Function1/1 -> Add1/1, Add/4
  Add1/1 -> Signed Sqrt/1
  Add/1 -> Divide/1
  Divide1/1 -> Trigonometric Function1/1
  Dot Product/1 -> Gain/1
  Add2/1 -> Divide1/1
  Gain/1 -> Divide1/2
  Divide/1 -> Trigonometric Function/1
  Trigonometric Function1/1 -> E/1
  Math Function2/1 -> Add2/1
  Math Function3/1 -> Add2/2
  Lower joint1/1 -> Math Function7/1, Dot Product/1
  Upper joint1/1 -> Dot Product/2, Math Function6/1
  Trigonometric Function/1 -> Add3/1
  Trigonometric Function2/1 -> Add3/2
  Add3/1 -> S/1
  Math Function5/1 -> Add/2
  Math Function4/1 -> Add/1
  Math Function7/1 -> Add2/3
  Math Function6/1 -> Add2/4
  Multiply/1 -> Divide/2
  Dot Product1/1 -> Multiply/1
  Signed Sqrt/1 -> Dot Product1/2
  Upper joint2/1 -> Dot Product1/1
  pi/2/1 -> Add3/3
  x/1 -> Multiply1/1
  Multiply1/1 -> Trigonometric Function2/2, Math Function/1, Math Function3/1

== system quadruped_2016/robot/FL/hip ==
  pos : Inport
  Rigid Transform1 : sm_lib/Frames and Transforms/Rigid Transform  TranslationMethod=StandardAxis  TranslationStandardOffset=Hip.gearboxCorrection  TranslationLengthUnit=mm  TranslationStandardAxis=-Z  TranslationCartesianOffset=50  TranslationROffset=0  TranslationROffsetUnits=m  TranslationZOffset=0  TranslationZOffsetUnits=m  TranslationThetaOffset=0  TranslationThetaOffsetUnits=deg  RotationMethod=None  RotationAngleUnits=deg  RotationStandardAxis=-X  RotationAngle=180  RotationArbitraryAxis=[0 0 1]  FollAlignAxisA=+X  BaseAlignAxisA=+Y  FollAlignAxisB=+Y  BaseAlignAxisB=+Z  RotationSequenceAxes=FollowerAxes  RotationSequence=XYZ  RotationSequenceAngles=[180 0 180]  RotationSequenceAnglesUnits=deg  RotationMatrix=[1 0 0; 0 1 0; 0 0 1]
  Rigid Transform6 : sm_lib/Frames and Transforms/Rigid Transform  TranslationMethod=Cartesian  TranslationStandardOffset=0.3  TranslationLengthUnit=mm  TranslationStandardAxis=+X  TranslationCartesianOffset=Hip.legGbxOft  TranslationROffset=0  TranslationROffsetUnits=m  TranslationZOffset=0  TranslationZOffsetUnits=m  TranslationThetaOffset=0  TranslationThetaOffsetUnits=deg  RotationMethod=StandardAxis  RotationAngleUnits=deg  RotationStandardAxis=-X  RotationAngle=90  RotationArbitraryAxis=[0 0 1]  FollAlignAxisA=+X  BaseAlignAxisA=+Y  FollAlignAxisB=+Y  BaseAlignAxisB=+Z  RotationSequenceAxes=FollowerAxes  RotationSequence=XYX  RotationSequenceAngles=[0 0 0]  RotationSequenceAnglesUnits=deg  RotationMatrix=[1 0 0; 0 1 0; 0 0 1]
  Rigid Transform7 : sm_lib/Frames and Transforms/Rigid Transform  TranslationMethod=Cartesian  TranslationStandardOffset=0.3  TranslationLengthUnit=mm  TranslationStandardAxis=+X  TranslationCartesianOffset=Hip.legOft  TranslationROffset=0  TranslationROffsetUnits=m  TranslationZOffset=0  TranslationZOffsetUnits=m  TranslationThetaOffset=0  TranslationThetaOffsetUnits=deg  RotationMethod=RotationSequence  RotationAngleUnits=deg  RotationStandardAxis=-X  RotationAngle=180  RotationArbitraryAxis=[0 0 1]  FollAlignAxisA=+X  BaseAlignAxisA=+Y  FollAlignAxisB=+Y  BaseAlignAxisB=+Z  RotationSequenceAxes=FollowerAxes  RotationSequence=XYZ  RotationSequenceAngles=[0 0 180]  RotationSequenceAnglesUnits=deg  RotationMatrix=[1 0 0; 0 1 0; 0 0 1]
  Rigid Transform8 : sm_lib/Frames and Transforms/Rigid Transform  TranslationMethod=Cartesian  TranslationStandardOffset=0.3  TranslationLengthUnit=mm  TranslationStandardAxis=+X  TranslationCartesianOffset=Hip.kneeGbxOft  TranslationROffset=0  TranslationROffsetUnits=m  TranslationZOffset=0  TranslationZOffsetUnits=m  TranslationThetaOffset=0  TranslationThetaOffsetUnits=deg  RotationMethod=StandardAxis  RotationAngleUnits=deg  RotationStandardAxis=-X  RotationAngle=90  RotationArbitraryAxis=[0 0 1]  FollAlignAxisA=+X  BaseAlignAxisA=+Y  FollAlignAxisB=+Y  BaseAlignAxisB=+Z  RotationSequenceAxes=FollowerAxes  RotationSequence=XYX  RotationSequenceAngles=[0 0 0]  RotationSequenceAnglesUnits=deg  RotationMatrix=[1 0 0; 0 1 0; 0 0 1]
  Sphere to Plane Force1 : Contact_Forces_Lib/3D/Sphere to Plane Force  sphere_rad=Leg.lower_joint.sphere_rad  plane_lenx=plane_dim(1)  plane_leny=plane_dim(2)  plane_depth=plane_dim(3)/2  force_law=Linear  k_contact=1e4  b_contact=1e2  pen_full_damp_F=1e-4  pen_exponent=1  custom_param_1=1  custom_param_2=1  friction_law=Stick-Slip Continuous  mu_kinetic=Leg.lower_joint.kine_frict  mu_static=Leg.lower_joint.stat_frict  v_thr=0.001  vis_on=off  vis_opc_en=0  vis_len_plaBz=0.005  vis_clr=[0.9 0.2 0.2]  vis_opc=0.7
  Terminator : Terminator
  hip motor : sm_lib/Body Elements/Solid  GraphicAmbientColor=[0.15 0.15 0.15 1.0]  BasedOnType=Mass  CenterOfMass=[0 0 0]  CenterOfMassUnits=m  GraphicDiffuseColor=Hip.GbxColor  CylinderLength=Hip.gearboxThickness  CylinderLengthUnits=mm  CylinderRadius=Hip.gearboxRadius  CylinderRadiusUnits=mm  Density=1000  DensityUnits=kg/m^3  DoExposeReferenceFrame=on  GraphicEmissiveColor=[0.0 0.0 0.0 1.0]  ExportEntireGeometry=off  SerializedFrames=<Frames/>  MarkerShape=Sphere  MarkerSize=10  GraphicType=FromGeometry  InertiaType=CalculateFromGeometry  Mass=Hip.gearboxMass  MassUnits=g  MomentsOfInertia=[1 1 1]  MomentsOfInertiaUnits=kg*m^2  GraphicOpacity=1.0  ProductsOfInertia=[0 0 0]  ProductsOfInertiaUnits=kg*m^2  GraphicShininess=75  GraphicSpecularColor=[0.5 0.5 0.5 1.0]  GraphicVisPropType=SimpleVisualProperties  GeometryShape=Cylinder
  joint : Subsystem  mask{Joint=Hip.joint}
  knee motor : sm_lib/Body Elements/Solid  GraphicAmbientColor=[0.15 0.15 0.15 1.0]  BasedOnType=Mass  CenterOfMass=[0 0 0]  CenterOfMassUnits=m  GraphicDiffuseColor=Hip.GbxColor  CylinderLength=Hip.gearboxThickness  CylinderLengthUnits=mm  CylinderRadius=Hip.gearboxRadius  CylinderRadiusUnits=mm  Density=1000  DensityUnits=kg/m^3  DoExposeReferenceFrame=on  GraphicEmissiveColor=[0.0 0.0 0.0 1.0]  ExportEntireGeometry=off  SerializedFrames=<Frames/>  MarkerShape=Sphere  MarkerSize=10  GraphicType=FromGeometry  InertiaType=CalculateFromGeometry  Mass=Hip.gearboxMass  MassUnits=g  MomentsOfInertia=[1 1 1]  MomentsOfInertiaUnits=kg*m^2  GraphicOpacity=1.0  ProductsOfInertia=[0 0 0]  ProductsOfInertiaUnits=kg*m^2  GraphicShininess=75  GraphicSpecularColor=[0.5 0.5 0.5 1.0]  GraphicVisPropType=SimpleVisualProperties  GeometryShape=Cylinder
  leg motor : sm_lib/Body Elements/Solid  GraphicAmbientColor=[0.15 0.15 0.15 1.0]  BasedOnType=Mass  CenterOfMass=[0 0 0]  CenterOfMassUnits=m  GraphicDiffuseColor=Hip.GbxColor  CylinderLength=Hip.gearboxThickness  CylinderLengthUnits=mm  CylinderRadius=Hip.gearboxRadius  CylinderRadiusUnits=mm  Density=1000  DensityUnits=kg/m^3  DoExposeReferenceFrame=on  GraphicEmissiveColor=[0.0 0.0 0.0 1.0]  ExportEntireGeometry=off  SerializedFrames=<Frames/>  MarkerShape=Sphere  MarkerSize=10  GraphicType=FromGeometry  InertiaType=CalculateFromGeometry  Mass=Hip.gearboxMass  MassUnits=g  MomentsOfInertia=[1 1 1]  MomentsOfInertiaUnits=kg*m^2  GraphicOpacity=1.0  ProductsOfInertia=[0 0 0]  ProductsOfInertiaUnits=kg*m^2  GraphicShininess=75  GraphicSpecularColor=[0.5 0.5 0.5 1.0]  GraphicVisPropType=SimpleVisualProperties  GeometryShape=Cylinder
  B : PMIOPort  Side=Left
  F : PMIOPort  Port=2  Side=Right
  plane : PMIOPort  Port=3  Side=Right
  p : Outport
  wires:
  Sphere to Plane Force1/1 -> Terminator/1
  pos/1 -> joint/1(in)
  joint/1(p) -> p/1
  connections:
  Rigid Transform7/RConn1 -- F/RConn1
  Rigid Transform6/RConn1 -- leg motor/RConn1 -- Rigid Transform7/LConn1
  Rigid Transform8/RConn1 -- knee motor/RConn1 -- Sphere to Plane Force1/LConn1
  Sphere to Plane Force1/RConn1 -- plane/RConn1
  B/RConn1 -- Rigid Transform1/LConn1
  joint/RConn1 -- Rigid Transform6/LConn1 -- Rigid Transform8/LConn1 -- hip motor/RConn1
  Rigid Transform1/RConn1 -- joint/LConn1

== system quadruped_2016/robot/FL/leg ==
  up pos : Inport
  lo pos : Inport  Port=2
  Bus Creator : BusCreator  Inputs=2
  Sphere to Plane Force1 : Contact_Forces_Lib/3D/Sphere to Plane Force  sphere_rad=Leg.lower_joint.sphere_rad  plane_lenx=plane_dim(1)  plane_leny=plane_dim(2)  plane_depth=plane_dim(3)/2  force_law=Linear  k_contact=1e4  b_contact=1e2  pen_full_damp_F=1e-4  pen_exponent=1  custom_param_1=1  custom_param_2=1  friction_law=Stick-Slip Continuous  mu_kinetic=Leg.lower_joint.kine_frict  mu_static=Leg.lower_joint.stat_frict  v_thr=0.001  vis_on=off  vis_opc_en=0  vis_len_plaBz=0.005  vis_clr=[0.9 0.2 0.2]  vis_opc=0.7
  Sphere to Plane Force2 : Contact_Forces_Lib/3D/Sphere to Plane Force  sphere_rad=Leg.lower_joint.sphere_rad  plane_lenx=plane_dim(1)  plane_leny=plane_dim(2)  plane_depth=plane_dim(3)/2  force_law=Linear  k_contact=1e4  b_contact=1e2  pen_full_damp_F=1e-4  pen_exponent=1  custom_param_1=1  custom_param_2=1  friction_law=Stick-Slip Continuous  mu_kinetic=Leg.lower_joint.kine_frict  mu_static=Leg.lower_joint.stat_frict  v_thr=0.001  vis_on=off  vis_opc_en=0  vis_len_plaBz=0.005  vis_clr=[0.9 0.2 0.2]  vis_opc=0.7
  Terminator : Terminator
  Terminator1 : Terminator
  Top2 : sm_lib/Frames and Transforms/Rigid Transform  TranslationMethod=StandardAxis  TranslationStandardOffset=Leg.lower_joint.sphere_rad  TranslationLengthUnit=m  TranslationStandardAxis=+X  TranslationCartesianOffset=[0 0 0.1]  TranslationROffset=0  TranslationROffsetUnits=m  TranslationZOffset=0  TranslationZOffsetUnits=m  TranslationThetaOffset=0  TranslationThetaOffsetUnits=deg  RotationMethod=None  RotationAngleUnits=deg  RotationStandardAxis=+Y  RotationAngle=90  RotationArbitraryAxis=[0 0 1]  FollAlignAxisA=+X  BaseAlignAxisA=+Y  FollAlignAxisB=+Y  BaseAlignAxisB=+Z  RotationSequenceAxes=FollowerAxes  RotationSequence=XYX  RotationSequenceAngles=[0 0 0]  RotationSequenceAnglesUnits=deg  RotationMatrix=[1 0 0; 0 1 0; 0 0 1]
  lower joint : Subsystem  mask{Leg_joint=Leg.lower_joint}
  upper joint : Subsystem  mask{Leg_joint=Leg.upper_joint}
  B : PMIOPort  Side=Left
  plane : PMIOPort  Port=2  Side=Right
  p : Outport
  wires:
  Sphere to Plane Force2/1 -> Terminator/1
  Sphere to Plane Force1/1 -> Terminator1/1
  up pos/1 -> upper joint/1(pos)
  lo pos/1 -> lower joint/1(pos)
  Bus Creator/1 -> p/1
  lower joint/1(p) -> Bus Creator/1  "lower joint data"
  upper joint/1(p) -> Bus Creator/2  "upper jount data"
  connections:
  Sphere to Plane Force2/LConn1 -- upper joint/RConn1 -- lower joint/LConn1
  upper joint/LConn1 -- B/RConn1
  Top2/LConn1 -- Sphere to Plane Force1/LConn1
  plane/RConn1 -- Sphere to Plane Force1/RConn1 -- Sphere to Plane Force2/RConn1
  lower joint/RConn1 -- Top2/RConn1

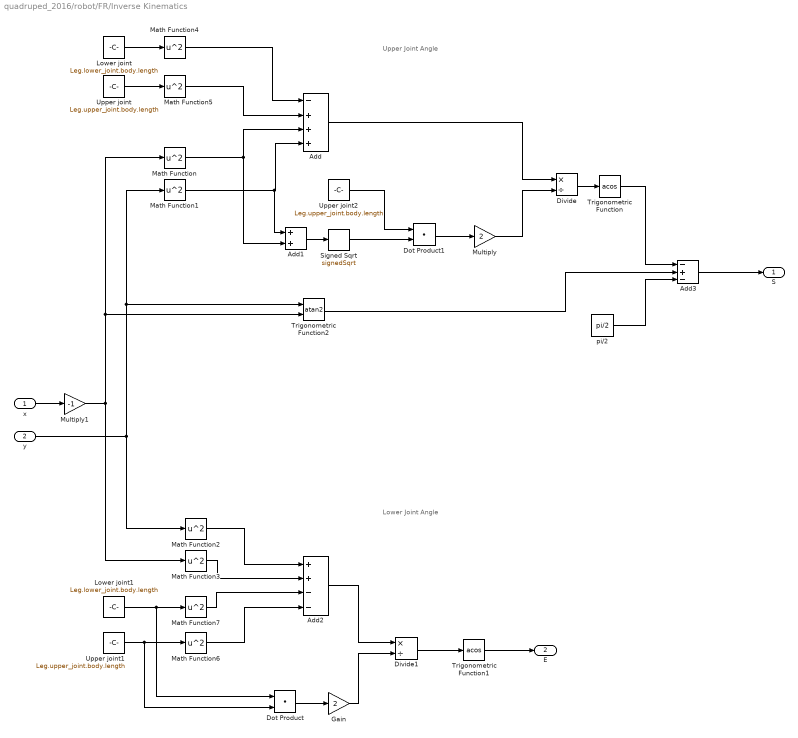
== system quadruped_2016/robot/FR/Inverse Kinematics  ==
  note: Upper Joint Angle
  note: Lower Joint Angle
  x : Inport
  y : Inport  Port=2
  Add : Sum  Inputs=-+++
  Add1 : Sum
  Add2 : Sum  Inputs=++--
  Add3 : Sum  Inputs=-+-
  Divide : Product  Inputs=*/
  Divide1 : Product  Inputs=*/
  Dot Product : DotProduct  InputSameDT=on  OutDataTypeStr=Inherit: Inherit via internal rule
  Dot Product1 : DotProduct  InputSameDT=on  OutDataTypeStr=Inherit: Inherit via internal rule
  Gain : Gain  Gain=2
  Lower joint : Constant  Value=Leg.lower_joint.body.length
  Lower joint1 : Constant  Value=Leg.lower_joint.body.length
  Math Function{,1..7} (8 alike) : Math  Operator=square  SaturateOnIntegerOverflow=on
  Multiply : Gain  Gain=2
  Multiply1 : Gain  Gain=-1
  Signed Sqrt : Sqrt  Operator=signedSqrt  SaturateOnIntegerOverflow=on
  Trigonometric Function : Trigonometry  Operator=acos
  Trigonometric Function1 : Trigonometry  Operator=acos
  Trigonometric Function2 : Trigonometry  Operator=atan2
  Upper joint : Constant  Value=Leg.upper_joint.body.length
  Upper joint1 : Constant  Value=Leg.upper_joint.body.length
  Upper joint2 : Constant  Value=Leg.upper_joint.body.length
  pi/2 : Constant  Value=pi/2
  S : Outport
  E : Outport  Port=2
  wires:
  y/1 -> Trigonometric Function2/1, Math Function1/1, Math Function2/1
  Lower joint/1 -> Math Function4/1
  Upper joint/1 -> Math Function5/1
  Math Function/1 -> Add1/2, Add/3
  Math Function1/1 -> Add1/1, Add/4
  Add1/1 -> Signed Sqrt/1
  Add/1 -> Divide/1
  Divide1/1 -> Trigonometric Function1/1
  Dot Product/1 -> Gain/1
  Add2/1 -> Divide1/1
  Gain/1 -> Divide1/2
  Divide/1 -> Trigonometric Function/1
  Trigonometric Function1/1 -> E/1
  Math Function2/1 -> Add2/1
  Math Function3/1 -> Add2/2
  Lower joint1/1 -> Math Function7/1, Dot Product/1
  Upper joint1/1 -> Dot Product/2, Math Function6/1
  Trigonometric Function/1 -> Add3/1
  Trigonometric Function2/1 -> Add3/2
  Add3/1 -> S/1
  Math Function5/1 -> Add/2
  Math Function4/1 -> Add/1
  Math Function7/1 -> Add2/3
  Math Function6/1 -> Add2/4
  Multiply/1 -> Divide/2
  Dot Product1/1 -> Multiply/1
  Signed Sqrt/1 -> Dot Product1/2
  Upper joint2/1 -> Dot Product1/1
  pi/2/1 -> Add3/3
  x/1 -> Multiply1/1
  Multiply1/1 -> Trigonometric Function2/2, Math Function/1, Math Function3/1
